simulink model "matlab_model"  (R2016b)
settings: Solver=VariableStepAuto  StartTime=0.0  StopTime=5  RelTol=1e-3
undefined symbols (not defined in the file): A, B, C, D, K_lqr, x0, xdesired
settings Model: Creator=r0610649  LastModifiedBy=r0610649

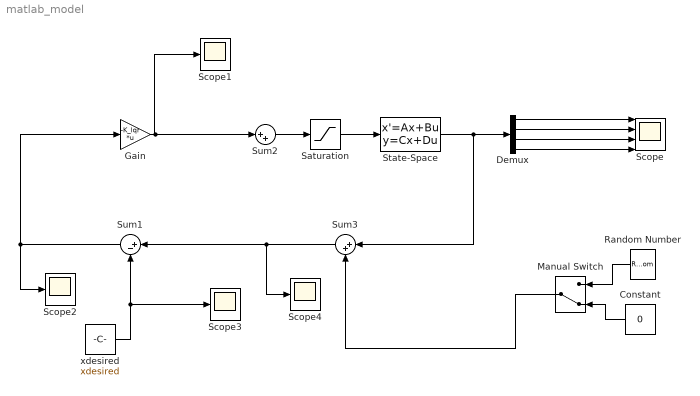
== system matlab_model ==
  Constant : Constant  Value=0
  Demux : Demux
  Gain : Gain  Gain=-K_lqr  Multiplication=Matrix(K*u)
  Manual Switch : ManualSwitch  CurrentSetting=0
  Random Number : RandomNumber  Variance=0.001  SampleTime=0.1
  Saturation : Saturate  UpperLimit=5  LowerLimit=-5
  Scope : Scope  NumInputPorts=4
  Scope{1..4} (4 alike) : Scope
  State-Space : StateSpace  A=A  B=B  C=C  D=D  X0=x0
  Sum1 : Sum  Inputs=|+-  OutMin=[2]  OutMax=[4]
  Sum2 : Sum  Inputs=|++
  Sum3 : Sum  Inputs=|++
  "xdesired " : Constant  Value=xdesired  SampleTime=.15
  wires:
  Saturation/1 -> State-Space/1
  State-Space/1 -> Sum3/1, Demux/1
  "xdesired "/1 -> Scope3/1, Sum1/2
  Sum1/1 -> Scope2/1, Gain/1
  Gain/1 -> Scope1/1, Sum2/1
  Demux/1 -> Scope/1
  Demux/2 -> Scope/2
  Demux/3 -> Scope/3
  Demux/4 -> Scope/4
  Sum2/1 -> Saturation/1
  Constant/1 -> Manual Switch/2
  Random Number/1 -> Manual Switch/1
  Manual Switch/1 -> Sum3/2
  Sum3/1 -> Scope4/1, Sum1/1
